simulink model "Modell_Diagnose"  (R2022a)
settings: Solver=FixedStepAuto  StartTime=0.0  StopTime=20.05  FixedStep=0.01  RelTol=1e-3
model workspace (MAT data in the model file):
  t_f = 7.2
libraries: simulink x3, fuzblock x1
settings Model: ParameterArgumentNames=t_f  Creator=Xueyong Lu  LastModifiedBy=Xueyong Lu

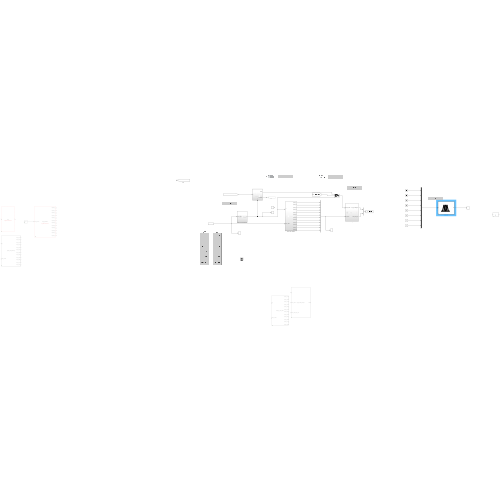
[thumbnail: Simulink's stored preview of the top-level diagram]
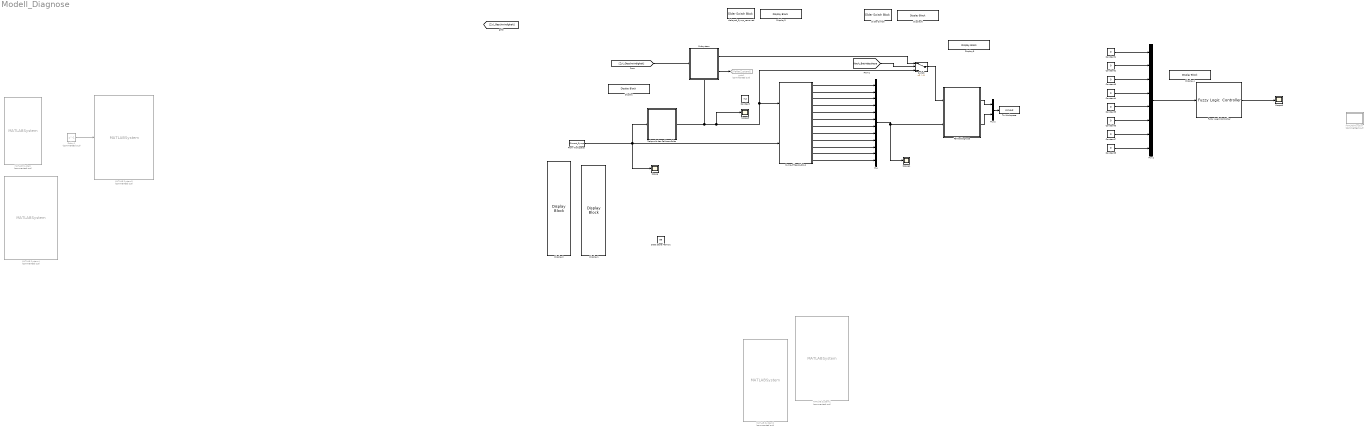
== system Modell_Diagnose ==
  Constant : Constant  Value=7.2  SampleTime=-1
  Constant{1..8} (8 alike) : Constant  Value=0
  Data Store Memory : DataStoreMemory  DataStoreName=aa  WriteAfterWriteMsg=warning  ShowAdditionalParam=off
  Delay1 : Delay  Commented=on  DelayLength=1
  Display{,3..6} (5 alike) : DisplayBlock  LabelPosition=Hide  Transparency=1
  Display1 : DisplayBlock  Transparency=1
  Display2 : DisplayBlock  Transparency=1  Layout=Fill available space
  Fehlerdiagnose : Subsystem
  From Workspace : FromWorkspace  VariableName=Simout_Symp  OutDataTypeStr=double  SampleTime=-1  OutputAfterFinalValue=Holding final value
  Fuzzy Logic Controller : fuzblock/Fuzzy Logic  Controller  FIS='Diagnose_fis_Still_Seite_A.fis'  OutputSampleNumber=101  DataType=double  FuzzifiedInputs=off  RuleFiringStrengths=off  RuleOutputs=off  AggregatedOutputs=off  SimulateUsing=Interpreted execution  OutOfRangeInputValueMessage=warning  NoRuleFiredMessage=warning  EmptyOutputFuzzySetMessage=warning
  MATLAB Function : MATLAB Function  Commented=on  TreatAsAtomicUnit=on
  MATLAB System : MATLABSystem  Commented=on  System=test  SimulateUsing=Code generation
      mask Type: test
      mask Display:
      | disp('test');
      | port_label('input',1,'u');
      | port_label('output',1,'y');
  MATLAB System1 : MATLABSystem  Commented=on  System=Symp_Filter_SubSys  SimulateUsing=Code generation
      mask Type: Symp_Filter_SubSys
      mask Display:
      | disp('Symp_Filter_SubSys');
      | port_label('input',1,'t_f');
      | port_label('input',2,'Time_series');
      | port_label('input',3,'Time_series_dis_der');
      | port_label('output',1,'Out');
  MATLAB System2 : MATLABSystem  Commented=on  System=output_in_eval_time  SimulateUsing=Code generation
      mask Type: output_in_eval_time
      mask Display:
      | disp('output_in_eval_time');
      | port_label('input',1,'t_f');
      | port_label('input',2,'Time_series');
      | port_label('output',1,'Symp_A1');
      | port_label('output',2,'Symp_A2');
      | port_label('output',3,'Symp_A3');
      | port_label('output',4,'Symp_A4');
      | port_label('output',5,'Symp_A5');
      | port_label('output',6,'Symp_B1');
      | port_label('output',7,'Symp_B2');
      | port_label('output',8,'Symp_B3');
      | port_label('output',9,'Symp_B4');
      | port_label('output',10,'Symp_B5');
      | port_label('output',11,'Symp_S1');
      | port_label('output',12,'Symp_S2');
  MATLAB System3 : MATLABSystem  Commented=on  System=Signal_Demux  SimulateUsing=Code generation
      mask Type: Signal_Demux
      mask Display:
      | disp('Signal_Demux');
      | port_label('input',1,'Time_series');
      | port_label('output',1,'Symp_A1');
      | port_label('output',2,'Symp_A2');
      | port_label('output',3,'Symp_A3');
      | port_label('output',4,'Symp_A4');
      | port_label('output',5,'Symp_A5');
      | port_label('output',6,'Symp_B1');
      | port_label('output',7,'Symp_B2');
      | port_label('output',8,'Symp_B3');
      | port_label('output',9,'Symp_B4');
      | port_label('output',10,'Symp_B5');
      | port_label('output',11,'Symp_S1');
      | port_label('output',12,'Symp_S2');
  MATLAB System4 : MATLABSystem  Commented=on  System=Symp_Filter_SubSys  SimulateUsing=Code generation
      mask Type: Symp_Filter_SubSys
      mask Display:
      | disp('Symp_Filter_SubSys');
      | port_label('input',1,'t_f');
      | port_label('input',2,'Time_series');
      | port_label('output',1,'Symp_A1');
      | port_label('output',2,'Symp_A2');
      | port_label('output',3,'Symp_A3');
      | port_label('output',4,'Symp_A4');
      | port_label('output',5,'Symp_A5');
      | port_label('output',6,'Symp_B1');
      | port_label('output',7,'Symp_B2');
      | port_label('output',8,'Symp_B3');
      | port_label('output',9,'Symp_B4');
      | port_label('output',10,'Symp_B5');
      | port_label('output',11,'Symp_S1');
      | port_label('output',12,'Symp_S2');
  Mux : Mux  Inputs=12
  Mux1 : Mux  Inputs=8
  Mux2 : Mux  Inputs=2
  Scope{,1,3,5} (4 alike) : Scope
  Slider Switch : SliderSwitchBlock
      settings: Values={{'Nach_t_f', 'Nach_vZyl'}, [0 1]}
  Subsystem : Subsystem
      settings: PortSchema="{\"entries\":[{\"content\":{\"sides\":[{\"content\":{\"connectorIds\":[\"In1\"]},\"type\":\"ConnectorPlacement.EquallySpacedRectSide\",\"uuid\":\"f9972d87-f39c-4f1f-a94a-1eb1a94210bf\"},{\"content\":{\"connectorIds\":[\"Out1\",\"Out2\"],\"side\":\"RIGHT\"},\"type\":\"ConnectorPlacement.EquallySpacedRectSide\",\"uuid\":\"518922ff-8880-4fb1-9f47-52b625cdf1df\"},{\"content\":{\"connectorIds\":[],\"side\":\"TOP\"},\"type\":\"ConnectorPlacement.EquallySpacedRectSide\",\"uuid\":\"62199aae-54b7-4722-ae08-096fbd9bf566\"},{\"content\":{\"connectorIds\":[\"In2\"],\"side\":\"BOTTOM\"},\"type\":\"ConnectorPlacement.EquallySpacedRectSide\",\"uuid\":\"39e1fdf6-478a-4c85-b443-9280ada7e399\"}]},\"type\":\"ConnectorPlacement.EquallySpacedConnector\",\"uuid\":\"c265ec14-a46e-406d-bb29-39e6e28d34ef\"}],\"packageUris\":[\"http://schema.mathworks.com/mf0/Connector/R2020b\"],\"version\":\"1.0\"}"
  Switch : Switch  Criteria=u2 > Threshold  SaturateOnIntegerOverflow=off  InputSameDT=off
  Symp_Filter_SubSys : Subsystem
  To Workspace : ToWorkspace  VariableName=simout  SaveFormat=Timeseries  SampleTime=-1
  Zeitpunkt des Fehlerauftritts : Subsystem
  delayed_Symp_removed : SliderSwitchBlock
      settings: Values={{'Off', 'On'}, [0 1]}
  goto1 : Goto  Commented=on  GotoTag=FehlerZustand
  wires:
  Symp_Filter_SubSys/1(Symp_A1) -> Mux/1
  Symp_Filter_SubSys/2(Symp_A2) -> Mux/2
  Symp_Filter_SubSys/3(Symp_A3) -> Mux/3
  Symp_Filter_SubSys/4(Symp_A4) -> Mux/4
  Symp_Filter_SubSys/5(Symp_A5) -> Mux/5
  Symp_Filter_SubSys/6(Symp_B1) -> Mux/6
  Symp_Filter_SubSys/7(Symp_B2) -> Mux/7
  Symp_Filter_SubSys/8(Symp_B3) -> Mux/8
  Symp_Filter_SubSys/9(Symp_B4) -> Mux/9
  Symp_Filter_SubSys/10(Symp_B5) -> Mux/10
  Symp_Filter_SubSys/11(Symp_S1) -> Mux/11
  Symp_Filter_SubSys/12(Symp_S2) -> Mux/12
  Delay1/1 -> MATLAB System3/1
  From Workspace/1 -> Zeitpunkt des Fehlerauftritts/1(Symp_matrix), Symp_Filter_SubSys/2(Symp_series), Scope/1
  Zeitpunkt des Fehlerauftritts/1(t_f) -> Subsystem/2(t_f), Scope3/1, Symp_Filter_SubSys/1(t_f), Switch/3
  Mux/1 -> Scope1/1, Fehlerdiagnose/2(Symptome)
  Constant8/1 -> Mux1/8
  Constant7/1 -> Mux1/7
  Constant6/1 -> Mux1/6
  Constant5/1 -> Mux1/5
  Constant4/1 -> Mux1/4
  Constant3/1 -> Mux1/3
  Constant2/1 -> Mux1/2
  Constant1/1 -> Mux1/1
  Mux1/1 -> Fuzzy Logic Controller/1
  Fuzzy Logic Controller/1 -> Scope5/1
  [Zyl_Geschwindigkeit] -> Subsystem/1(In1)
  Subsystem/2(FaultState) -> goto1/1
  Switch/1 -> Fehlerdiagnose/1(Fehler_Phase)
  [Nach_Betriebsphase] -> Switch/2
  Subsystem/1(Phase) -> Switch/1
  Fehlerdiagnose/1(Symp_zurDiagnose) -> Mux2/1
  Fehlerdiagnose/2(Fehler_komp_Nr) -> Mux2/2
  Mux2/1 -> To Workspace/1

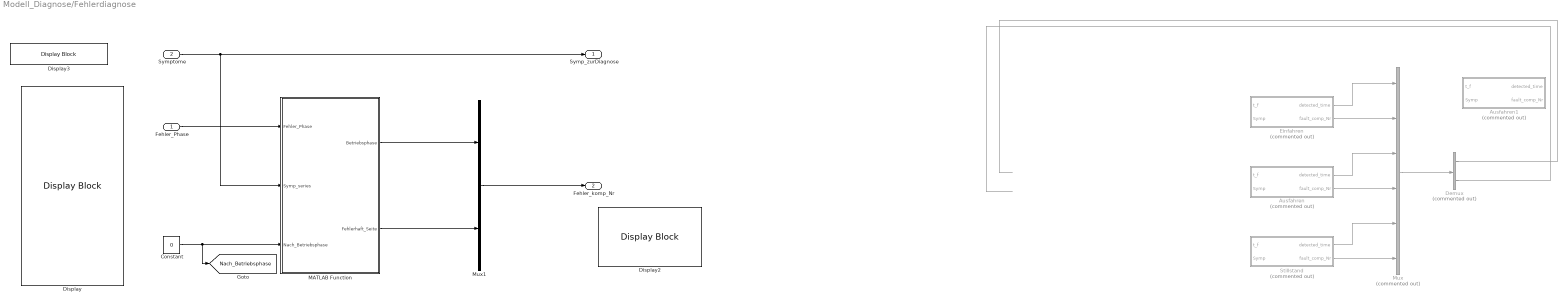
== system Modell_Diagnose/Fehlerdiagnose ==
  Fehler_Phase : Inport
  Symptome : Inport  Port=2
  Ausfahren : Subsystem  Commented=on
  Ausfahren1 : Subsystem  Commented=on
  Constant : Constant  Value=0
  Demux : Demux  Commented=on  Outputs=2
  Display : DisplayBlock  LabelPosition=Hide  Format=long  Transparency=1  Layout=Fill available space
  Display2 : DisplayBlock  LabelPosition=Hide  Transparency=1
  Display3 : DisplayBlock  LabelPosition=Hide  Transparency=1
  Einfahren : Subsystem  Commented=on
  MATLAB Function : MATLAB Function  TreatAsAtomicUnit=on
  Mux : Mux  Commented=on  Inputs=6
  Mux1 : Mux  Inputs=2
  Stillstand : Subsystem  Commented=on
  Symp_zurDiagnose : Outport
  Fehler_komp_Nr : Outport  Port=2
  tag scope: Nach_Betriebsphase=global
  wires:
  ? -> Einfahren/1(t_f)
  ? -> Ausfahren/1(t_f)
  ? -> Stillstand/1(t_f)
  Einfahren/1(detected_time) -> Mux/1
  Mux/1 -> Demux/1
  Einfahren/2(fault_comp_Nr) -> Mux/2
  Ausfahren/1(detected_time) -> Mux/3
  Ausfahren/2(fault_comp_Nr) -> Mux/4
  Stillstand/1(detected_time) -> Mux/5
  Stillstand/2(fault_comp_Nr) -> Mux/6
  Demux/1 -> ?
  Demux/2 -> ?
  Constant/1 -> MATLAB Function/3(Nach_Betriebsphase), [Nach_Betriebsphase]
  Fehler_Phase/1 -> MATLAB Function/1(Fehler_Phase)
  Mux1/1 -> Fehler_komp_Nr/1
  Symptome/1 -> MATLAB Function/2(Symp_series), Symp_zurDiagnose/1
  MATLAB Function/1(Betriebsphase) -> Mux1/1
  MATLAB Function/2(Fehlerhaft_Seite) -> Mux1/2

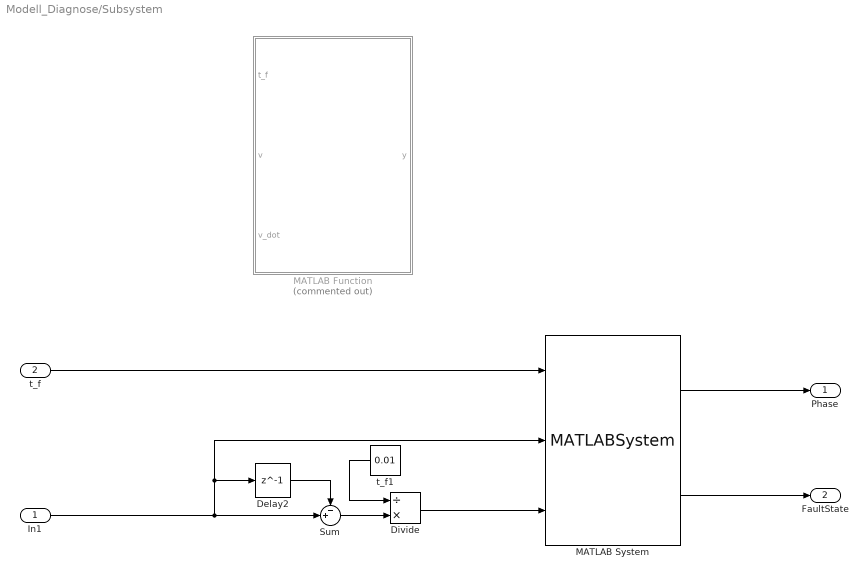
== system Modell_Diagnose/Subsystem ==
  In1 : Inport
  t_f : Inport  Port=2
  Delay2 : Delay  DelayLength=1
  Divide : Product  Inputs=/*
  MATLAB Function : MATLAB Function  Commented=on  TreatAsAtomicUnit=on
  MATLAB System : MATLABSystem  System=Betriebs_Phase  SimulateUsing=Code generation
      mask Type: Betriebs_Phase
      mask Display:
      | disp('Betriebs_Phase');
      | port_label('input',1,'t_f');
      | port_label('input',2,'v');
      | port_label('input',3,'v_dot');
      | port_label('output',1,'Phase');
      | port_label('output',2,'Fault_State');
  Sum : Sum  Inputs=-+|
  t_f1 : Constant  Value=0.01  VectorParams1D=off
  Phase : Outport
  FaultState : Outport  Port=2
  wires:
  In1/1 -> MATLAB System/2, Delay2/1, Sum/2
  t_f1/1 -> Divide/1
  Sum/1 -> Divide/2
  Delay2/1 -> Sum/1
  Divide/1 -> MATLAB System/3
  t_f/1 -> MATLAB System/1
  MATLAB System/1 -> Phase/1
  MATLAB System/2 -> FaultState/1

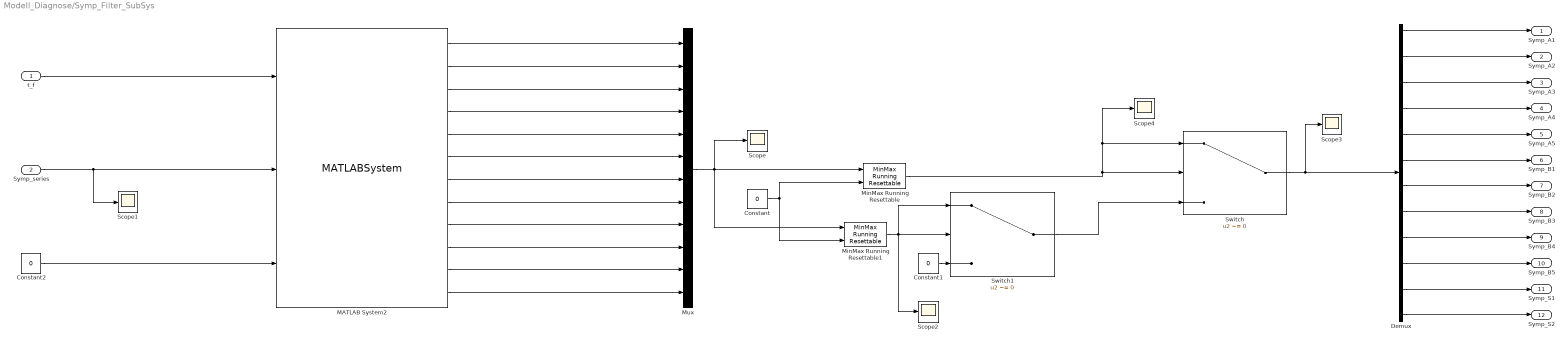
== system Modell_Diagnose/Symp_Filter_SubSys ==
  t_f : Inport
  Symp_series : Inport  Port=2
  Constant : Constant  Value=0  OutDataTypeStr=boolean
  Constant1 : Constant  Value=0  OutDataTypeStr=boolean
  Constant2 : Constant  Value=0
  Demux : Demux  Outputs=12
  MATLAB System2 : MATLABSystem  System=output_in_eval_time  SimulateUsing=Code generation
      mask Type: output_in_eval_time
      mask Display:
      | disp('output_in_eval_time');
      | port_label('input',1,'t_f');
      | port_label('input',2,'Symp_series');
      | port_label('input',3,'delayed_Symp_removed');
      | port_label('output',1,'Symp_A1');
      | port_label('output',2,'Symp_A2');
      | port_label('output',3,'Symp_A3');
      | port_label('output',4,'Symp_A4');
      | port_label('output',5,'Symp_A5');
      | port_label('output',6,'Symp_B1');
      | port_label('output',7,'Symp_B2');
      | port_label('output',8,'Symp_B3');
      | port_label('output',9,'Symp_B4');
      | port_label('output',10,'Symp_B5');
      | port_label('output',11,'Symp_S1');
      | port_label('output',12,'Symp_S2');
  MinMax Running Resettable : simulink/Math Operations/MinMax Running Resettable  Function=max  vinit=0.0
  MinMax Running Resettable1 : simulink/Math Operations/MinMax Running Resettable  Function=min  vinit=0.0
  Mux : Mux  Inputs=12
  Scope{,1..4} (5 alike) : Scope
  Switch : Switch  Criteria=u2 ~= 0  SaturateOnIntegerOverflow=off  InputSameDT=off
  Switch1 : Switch  Criteria=u2 ~= 0  SaturateOnIntegerOverflow=off  InputSameDT=off
  Symp_A1 : Outport
  Symp_A2 : Outport  Port=2
  Symp_A3 : Outport  Port=3
  Symp_A4 : Outport  Port=4
  Symp_A5 : Outport  Port=5
  Symp_B1 : Outport  Port=6
  Symp_B2 : Outport  Port=7
  Symp_B3 : Outport  Port=8
  Symp_B4 : Outport  Port=9
  Symp_B5 : Outport  Port=10
  Symp_S1 : Outport  Port=11
  Symp_S2 : Outport  Port=12
  wires:
  Symp_series/1 -> Scope1/1, MATLAB System2/2
  MATLAB System2/1 -> Mux/1
  MATLAB System2/2 -> Mux/2
  MATLAB System2/3 -> Mux/3
  MATLAB System2/4 -> Mux/4
  MATLAB System2/5 -> Mux/5
  MATLAB System2/6 -> Mux/6
  MATLAB System2/7 -> Mux/7
  MATLAB System2/8 -> Mux/8
  MATLAB System2/9 -> Mux/9
  MATLAB System2/10 -> Mux/10
  MATLAB System2/11 -> Mux/11
  MATLAB System2/12 -> Mux/12
  MinMax Running Resettable1/1 -> Scope2/1, Switch1/1, Switch1/2
  Switch/1 -> Scope3/1, Demux/1
  Mux/1 -> Scope/1, MinMax Running Resettable/1, MinMax Running Resettable1/1
  MinMax Running Resettable/1 -> Switch/1, Scope4/1, Switch/2
  Constant/1 -> MinMax Running Resettable1/2, MinMax Running Resettable/2
  Switch1/1 -> Switch/3
  Constant1/1 -> Switch1/3
  Demux/1 -> Symp_A1/1
  Demux/2 -> Symp_A2/1
  Demux/3 -> Symp_A3/1
  Demux/4 -> Symp_A4/1
  Demux/5 -> Symp_A5/1
  Demux/6 -> Symp_B1/1
  Demux/7 -> Symp_B2/1
  Demux/8 -> Symp_B3/1
  Demux/9 -> Symp_B4/1
  Demux/10 -> Symp_B5/1
  Demux/11 -> Symp_S1/1
  Demux/12 -> Symp_S2/1
  t_f/1 -> MATLAB System2/1
  Constant2/1 -> MATLAB System2/3

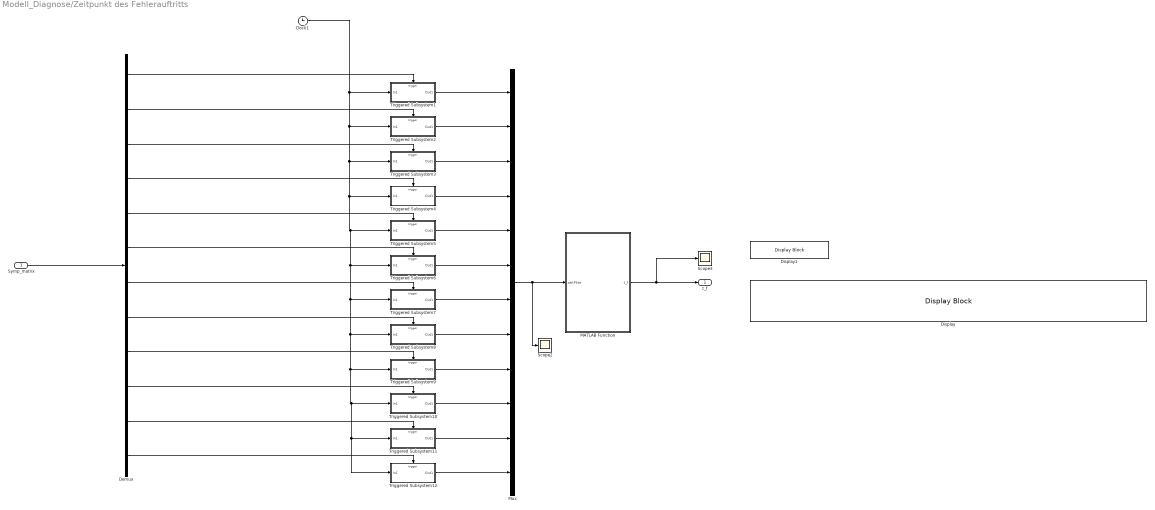
== system Modell_Diagnose/Zeitpunkt des Fehlerauftritts ==
  Symp_matrix : Inport
  Clock1 : Clock
  Demux : Demux  Outputs=12
  Display : DisplayBlock  LabelPosition=Hide  Transparency=1
  Display1 : DisplayBlock  LabelPosition=Hide  Transparency=1
  MATLAB Function : MATLAB Function  TreatAsAtomicUnit=on
  Mux : Mux  Inputs=12
  Scope2 : Scope
  Scope3 : Scope
  Triggered Subsystem1 : Subsystem  TreatAsAtomicUnit=on
  Triggered Subsystem10 : Subsystem  TreatAsAtomicUnit=on
  Triggered Subsystem11 : Subsystem  TreatAsAtomicUnit=on
  Triggered Subsystem12 : Subsystem  TreatAsAtomicUnit=on
  Triggered Subsystem2 : Subsystem  TreatAsAtomicUnit=on
  Triggered Subsystem3 : Subsystem  TreatAsAtomicUnit=on
  Triggered Subsystem4 : Subsystem  TreatAsAtomicUnit=on
  Triggered Subsystem5 : Subsystem  TreatAsAtomicUnit=on
  Triggered Subsystem6 : Subsystem  TreatAsAtomicUnit=on
  Triggered Subsystem7 : Subsystem  TreatAsAtomicUnit=on
  Triggered Subsystem8 : Subsystem  TreatAsAtomicUnit=on
  Triggered Subsystem9 : Subsystem  TreatAsAtomicUnit=on
  t_f : Outport
  wires:
  Demux/2 -> Triggered Subsystem2/Trigger
  Demux/1 -> Triggered Subsystem1/Trigger
  Demux/3 -> Triggered Subsystem3/Trigger
  Demux/4 -> Triggered Subsystem4/Trigger
  Demux/6 -> Triggered Subsystem6/Trigger
  Demux/5 -> Triggered Subsystem5/Trigger
  Demux/7 -> Triggered Subsystem7/Trigger
  Clock1/1 -> Triggered Subsystem4/1(In1), Triggered Subsystem12/1(In1), Triggered Subsystem11/1(In1), Triggered Subsystem10/1(In1), Triggered Subsystem9/1(In1), Triggered Subsystem8/1(In1), Triggered Subsystem7/1(In1), Triggered Subsystem6/1(In1), Triggered Subsystem5/1(In1), Triggered Subsystem3/1(In1), Triggered Subsystem2/1(In1), Triggered Subsystem1/1(In1)
  Triggered Subsystem1/1(Out1) -> Mux/1
  Symp_matrix/1 -> Demux/1
  Mux/1 -> Scope2/1, MATLAB Function/1(zeitPkte)
  MATLAB Function/1(t_f) -> Scope3/1, t_f/1
  Demux/8 -> Triggered Subsystem8/Trigger
  Demux/9 -> Triggered Subsystem9/Trigger
  Demux/10 -> Triggered Subsystem10/Trigger
  Demux/11 -> Triggered Subsystem11/Trigger
  Demux/12 -> Triggered Subsystem12/Trigger
  Triggered Subsystem12/1(Out1) -> Mux/12
  Triggered Subsystem2/1(Out1) -> Mux/2
  Triggered Subsystem3/1(Out1) -> Mux/3
  Triggered Subsystem4/1(Out1) -> Mux/4
  Triggered Subsystem5/1(Out1) -> Mux/5
  Triggered Subsystem6/1(Out1) -> Mux/6
  Triggered Subsystem7/1(Out1) -> Mux/7
  Triggered Subsystem8/1(Out1) -> Mux/8
  Triggered Subsystem9/1(Out1) -> Mux/9
  Triggered Subsystem10/1(Out1) -> Mux/10
  Triggered Subsystem11/1(Out1) -> Mux/11

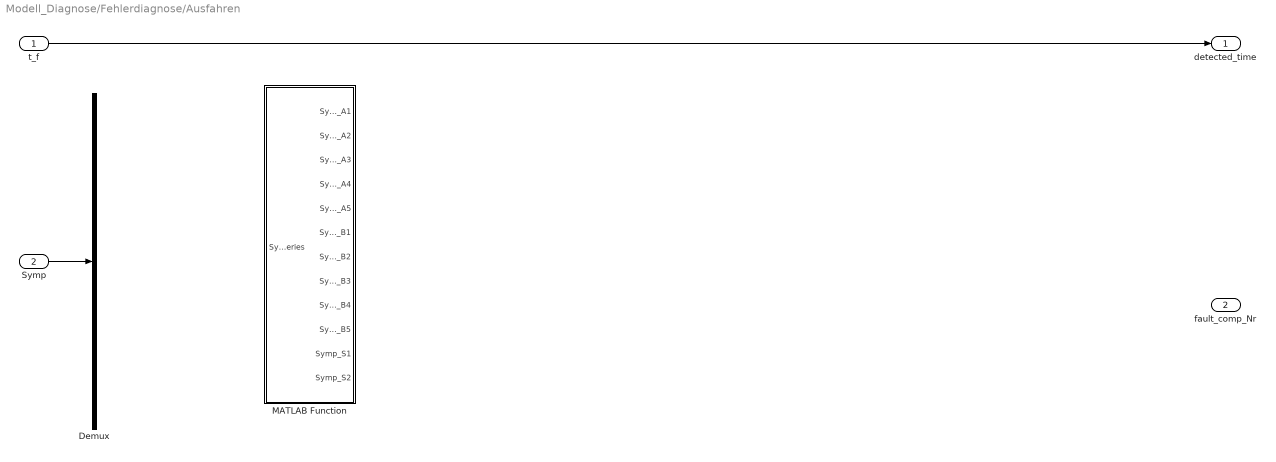
== system Modell_Diagnose/Fehlerdiagnose/Ausfahren ==
  t_f : Inport
  Symp : Inport  Port=2
  Demux : Demux  Outputs=12
  MATLAB Function : MATLAB Function  TreatAsAtomicUnit=on
  detected_time : Outport
  fault_comp_Nr : Outport  Port=2
  wires:
  Symp/1 -> Demux/1
  t_f/1 -> detected_time/1

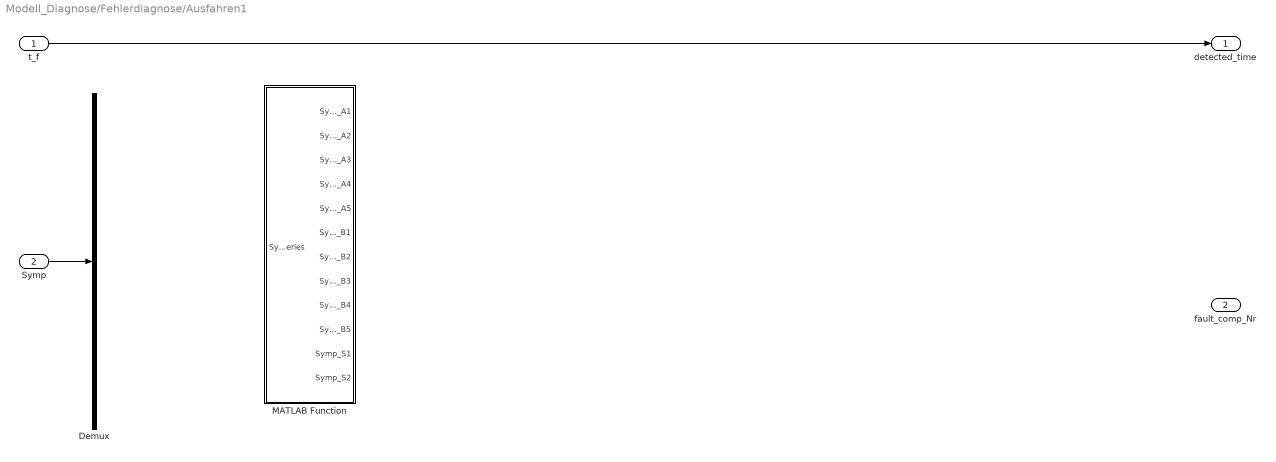
== system Modell_Diagnose/Fehlerdiagnose/Ausfahren1 ==
  t_f : Inport
  Symp : Inport  Port=2
  Demux : Demux  Outputs=12
  MATLAB Function : MATLAB Function  TreatAsAtomicUnit=on
  detected_time : Outport
  fault_comp_Nr : Outport  Port=2
  wires:
  Symp/1 -> Demux/1
  t_f/1 -> detected_time/1

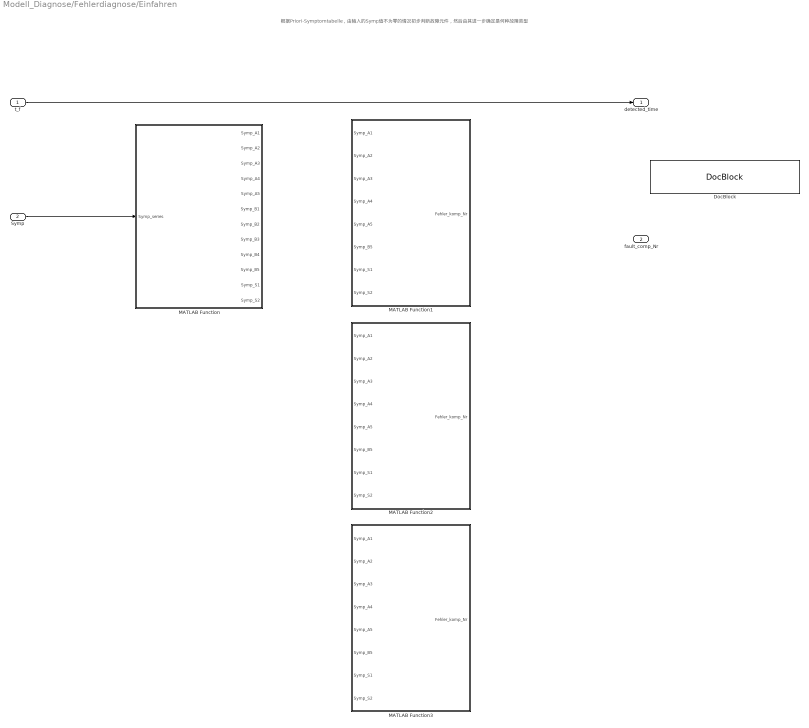
== system Modell_Diagnose/Fehlerdiagnose/Einfahren ==
  note: 根据Priori-Symptomtabelle，由输入的Symp值不为零的情况初步判断故障元件，然后由其进一步确定是何种故障类型
  t_f : Inport
  Symp : Inport  Port=2
  DocBlock : simulink/Model-Wide Utilities/DocBlock  DocumentType=Text
      content=|
      | 根据Priori-Symptomtabelle，由输入的Symp值不为零的情况初步判断故障元件，然后由其进一步确定是何种故障类型
  MATLAB Function : MATLAB Function  TreatAsAtomicUnit=on
  MATLAB Function1 : MATLAB Function  TreatAsAtomicUnit=on
  MATLAB Function2 : MATLAB Function  TreatAsAtomicUnit=on
  MATLAB Function3 : MATLAB Function  TreatAsAtomicUnit=on
  detected_time : Outport
  fault_comp_Nr : Outport  Port=2
  wires:
  Symp/1 -> MATLAB Function/1(Symp_series)
  t_f/1 -> detected_time/1

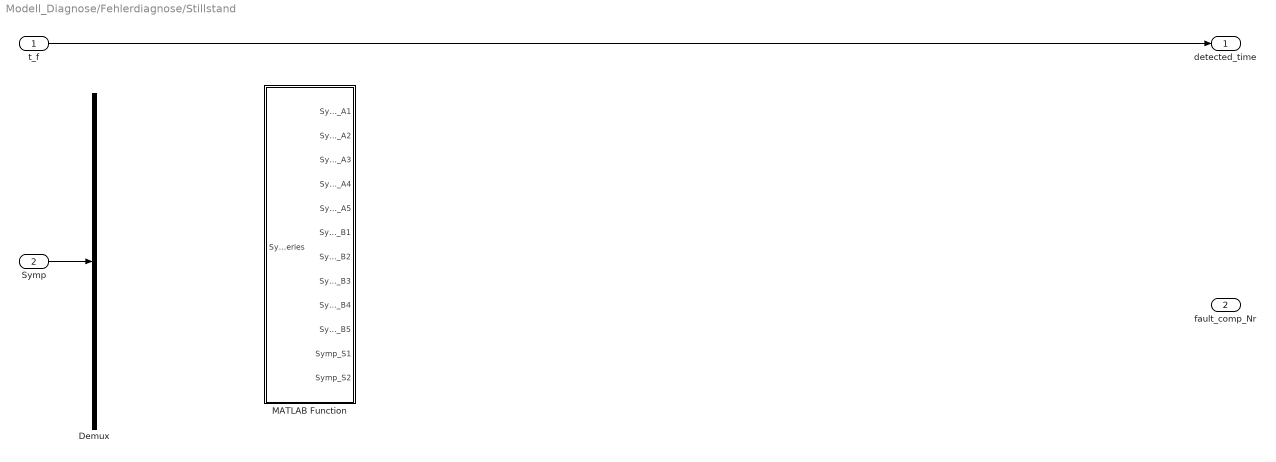
== system Modell_Diagnose/Fehlerdiagnose/Stillstand ==
  t_f : Inport
  Symp : Inport  Port=2
  Demux : Demux  Outputs=12
  MATLAB Function : MATLAB Function  TreatAsAtomicUnit=on
  detected_time : Outport
  fault_comp_Nr : Outport  Port=2
  wires:
  Symp/1 -> Demux/1
  t_f/1 -> detected_time/1

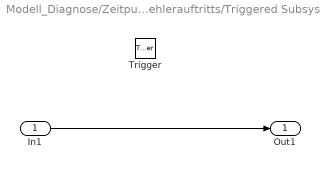
== system Modell_Diagnose/Zeitpunkt des Fehlerauftritts/Triggered Subsystem1 ==
  In1 : Inport
  Trigger : TriggerPort  TriggerType=either  VariantControl=(inherit)
  Out1 : Outport
  wires:
  In1/1 -> Out1/1

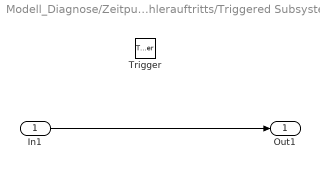
== system Modell_Diagnose/Zeitpunkt des Fehlerauftritts/Triggered Subsystem10 ==
  In1 : Inport
  Trigger : TriggerPort  TriggerType=either  VariantControl=(inherit)
  Out1 : Outport
  wires:
  In1/1 -> Out1/1

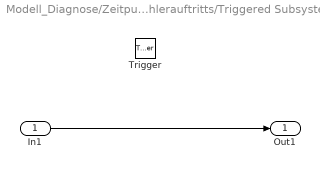
== system Modell_Diagnose/Zeitpunkt des Fehlerauftritts/Triggered Subsystem11 ==
  In1 : Inport
  Trigger : TriggerPort  TriggerType=either  VariantControl=(inherit)
  Out1 : Outport
  wires:
  In1/1 -> Out1/1

== system Modell_Diagnose/Zeitpunkt des Fehlerauftritts/Triggered Subsystem12 ==
  In1 : Inport
  Trigger : TriggerPort  TriggerType=either  VariantControl=(inherit)
  Out1 : Outport
  wires:
  In1/1 -> Out1/1

== system Modell_Diagnose/Zeitpunkt des Fehlerauftritts/Triggered Subsystem2 ==
  In1 : Inport
  Trigger : TriggerPort  TriggerType=either  VariantControl=(inherit)
  Out1 : Outport
  wires:
  In1/1 -> Out1/1

== system Modell_Diagnose/Zeitpunkt des Fehlerauftritts/Triggered Subsystem3 ==
  In1 : Inport
  Trigger : TriggerPort  TriggerType=either  VariantControl=(inherit)
  Out1 : Outport
  wires:
  In1/1 -> Out1/1

== system Modell_Diagnose/Zeitpunkt des Fehlerauftritts/Triggered Subsystem4 ==
  In1 : Inport
  Trigger : TriggerPort  TriggerType=either  VariantControl=(inherit)
  Out1 : Outport
  wires:
  In1/1 -> Out1/1

== system Modell_Diagnose/Zeitpunkt des Fehlerauftritts/Triggered Subsystem5 ==
  In1 : Inport
  Trigger : TriggerPort  TriggerType=either  VariantControl=(inherit)
  Out1 : Outport
  wires:
  In1/1 -> Out1/1

== system Modell_Diagnose/Zeitpunkt des Fehlerauftritts/Triggered Subsystem6 ==
  In1 : Inport
  Trigger : TriggerPort  TriggerType=either  VariantControl=(inherit)
  Out1 : Outport
  wires:
  In1/1 -> Out1/1

== system Modell_Diagnose/Zeitpunkt des Fehlerauftritts/Triggered Subsystem7 ==
  In1 : Inport
  Trigger : TriggerPort  TriggerType=either  VariantControl=(inherit)
  Out1 : Outport
  wires:
  In1/1 -> Out1/1

== system Modell_Diagnose/Zeitpunkt des Fehlerauftritts/Triggered Subsystem8 ==
  In1 : Inport
  Trigger : TriggerPort  TriggerType=either  VariantControl=(inherit)
  Out1 : Outport
  wires:
  In1/1 -> Out1/1

== system Modell_Diagnose/Zeitpunkt des Fehlerauftritts/Triggered Subsystem9 ==
  In1 : Inport
  Trigger : TriggerPort  TriggerType=either  VariantControl=(inherit)
  Out1 : Outport
  wires:
  In1/1 -> Out1/1

== matlab function Modell_Diagnose/Fehlerdiagnose/Einfahren/MATLAB Function1 ==
  data: Fehler_komp_Nr output; Symp_A1 input; Symp_A2 input; Symp_A3 input; Symp_A4 input; Symp_A5 input; Symp_B5 input; Symp_S1 input; Symp_S2 input
function Fehler_komp_Nr = Einfahren_Seite_A(Symp_A1,Symp_A2,Symp_A3,Symp_A4,Symp_A5,Symp_B5,Symp_S1,Symp_S2)

== matlab function Modell_Diagnose/Fehlerdiagnose/Einfahren/MATLAB Function2 ==
  data: Fehler_komp_Nr output; Symp_A1 input; Symp_A2 input; Symp_A3 input; Symp_A4 input; Symp_A5 input; Symp_B5 input; Symp_S1 input; Symp_S2 input
function Fehler_komp_Nr = Einfahren_Seite_B(Symp_A1,Symp_A2,Symp_A3,Symp_A4,Symp_A5,Symp_B5,Symp_S1,Symp_S2)

== matlab function Modell_Diagnose/Fehlerdiagnose/Einfahren/MATLAB Function3 ==
  data: Fehler_komp_Nr output; Symp_A1 input; Symp_A2 input; Symp_A3 input; Symp_A4 input; Symp_A5 input; Symp_B5 input; Symp_S1 input; Symp_S2 input
function Fehler_komp_Nr = Einfahren_Seite_S(Symp_A1,Symp_A2,Symp_A3,Symp_A4,Symp_A5,Symp_B5,Symp_S1,Symp_S2)

== matlab function Modell_Diagnose/Fehlerdiagnose/Ausfahren1/MATLAB Function ==
  data: Symp_A1 output; Symp_series input; Symp_A2 output; Symp_A3 output; Symp_A4 output; Symp_A5 output; Symp_B1 output; Symp_B2 output; Symp_B3 output; Symp_B4 output; Symp_B5 output; Symp_S1 output; Symp_S2 output
function [Symp_A1,Symp_A2,Symp_A3,Symp_A4,Symp_A5,Symp_B1,Symp_B2,Symp_B3,Symp_B4,Symp_B5,Symp_S1,Symp_S2] = fcn(Symp_series)
    
y = u;

== matlab function Modell_Diagnose/Subsystem/MATLAB Function ==
  data: t_f input; v input; y output; v_dot input
function y = Betriebs_Phase1(t_f,v,v_dot)
    if v < 0
        if v_dot < 0
            y = 1;
        elseif v_dot == 0
            y = 2;
        else 
            y = 3;
        end
    elseif v > 0
        if v_dot > 0
            y = 5;
        elseif v_dot == 0
            y = 6;
        else
            y=7;
        end
    else
        if v_dot == 0
            y = 4;
        end
    end

== matlab function Modell_Diagnose/Fehlerdiagnose/MATLAB Function ==
  settings: updateMethod=DISCRETE
  data: Betriebsphase output; Fehlerhaft_Seite output; Fehler_Phase input; Symp_series input; Nach_Betriebsphase input
function [Betriebsphase,Fehlerhaft_Seite] = fcn(Fehler_Phase,Symp_series,Nach_Betriebsphase)
%% Ermittlung der Betriebsphase des Fehlerauftritts
Betriebsphase = nan;  % Initialisierung der Ausgangsgrößen
Fehlerhaft_Seite = nan;

if logical(Nach_Betriebsphase)
%     case 1
        if Fehler_Phase == 1 || Fehler_Phase == 2 || Fehler_Phase == 3
            Betriebsphase = 1; % Einfahren
        elseif Fehler_Phase == 5 || Fehler_Phase == 6 || Fehler_Phase == 7
            Betriebsphase = 2; % Ausfahren
        elseif Fehler_Phase == 4
            Betriebsphase = 3; % Stillstand
        end
%     case 0
else
        if Fehler_Phase < 12
            Betriebsphase = 1; % Einfahren
        elseif Fehler_Phase > 14 && Fehler_Phase < 20
            Betriebsphase = 2; % Ausfahren
        elseif Fehler_Phase == 20
            Betriebsphase = 0;
        else
            Betriebsphase = 3; % Stillstand
        end
end
%% Lokalisierung der fehlerhaften Seite
switch Betriebsphase
    %% Phase der Fehlererkennung: Einfahren
    % A:1, B:2, S:3, unerkennbar A-P,B-T: 4, unerkennbar A-T, B-P: 5 
    case 1
    if all(Symp_series==0)
        Fehlerhaft_Seite = 0;

    elseif all(Symp_series(1:9)==0)   % A1-B4
        if Symp_series(10)==0         % B5 == 0
            if all(Symp_series(11:12) < 0)  % S1-S2
                Fehlerhaft_Seite = 1; % A-P_min
            elseif all(Symp_series(11:12) > 0)
                Fehlerhaft_Seite = 5; % A-T_max, B-P_max, p0_sens
            elseif Symp_series(11)<0 && Symp_series(12)==0
                Fehlerhaft_Seite = 1; % pA_sens
            elseif Symp_series(11) == 0 && Symp_series(12) > 0
                Fehlerhaft_Seite = 3; % p0_sens
            end
        elseif Symp_series(10) > 0    % B5 > 0
            if all(Symp_series(11:12) < 0)
                Fehlerhaft_Seite = 4; % A-P_max, B-T_max
            elseif all(Symp_series(11:12) == 0)
                Fehlerhaft_Seite = 2; % B-T_max
            end
        elseif Symp_series(10) < 0    % B5 < 0
            if all(Symp_series(11:12) > 0)
                Fehlerhaft_Seite = 3; % p0_sens
            end
        end

    elseif length(find(Symp_series(1:5)~=0)) > length(find(Symp_series(6:10)~=0))...
            && length(find(Symp_series(6:10)~=0))<=1                       % Symptome auf der Seite_A > die auf der Seite_B
        [A_NonNull_Nr,NonNull_ind] = find(Symp_series(1:5)~=0);
        switch length(A_NonNull_Nr)
            case 1
                if NonNull_ind(1) == 1
                    if all(Symp_series(2:12) == 0)
                        Fehlerhaft_Seite = 6; % --> swA-T, p0_sens, pT_sens; Eintragen in Seite S
                    else 
                        Fehlerhaft_Seite = 3;
                    end
                elseif NonNull_ind(1) == 4
                    if ~all(Symp_series(2:12) == 0)
                        Fehlerhaft_Seite = 3; % vZyl
                    else
                        Fehlerhaft_Seite = 1;
                    end
                else
                    Fehlerhaft_Seite = 1;
                end

            case 2 
                if all(NonNull_ind == [1 4])
                    Fehlerhaft_Seite = 3; % vZyl_sens
                elseif all(NonNull_ind == [3 4])
                    Fehlerhaft_Seite = 7; % vZyl_sens, pGSK_A, p_A_sens --> Eintragen in Seite A
                else
                    Fehlerhaft_Seite = 1;
%                     Symp_Vektor = Symp_series([1:5 10 11:12]);
                end

            case 3
                if all(NonNull_ind == [1 3 4])
                    Fehlerhaft_Seite = 8; % vZyl_sens, pA_sens --> Eintragen in Seite A (1)
                else
                    Fehlerhaft_Seite = 1;
                end

            case 4
                Fehlerhaft_Seite = 1;
        end

%         Symp_Vektor = Symp_series()
    
    elseif length(find(Symp_series(1:5)~=0)) <= length(find(Symp_series(6:10)~=0))...
            && length(find(Symp_series(1:5)~=0))<=1                       % Symptome auf der Seite_B >= die auf der Seite_A

        [A_NonNull_Nr,NonNull_ind] = find(Symp_series(6:10)~=0);
        switch length(A_NonNull_Nr)
            case 1
                if NonNull_ind(1) == 6
                    if all(Symp_series([1:5 11:12])==0)
                        Fehlerhaft_Seite = 8; % p0_sens, sw_B-P_min --> Eintragen in Seite B (2)
                    elseif Symp_series(1)~=0
                        Fehlerhaft_Seite = 1;
                    else
                        Fehlerhaft_Seite = 3;
                    end
                elseif NonNull_ind(1) == 10
                    if all(Symp_series(1:5)==0)
                        Fehlerhaft_Seite = 3;
                    else
                        Fehlerhaft_Seite = 2;
                    end
                end

            case 2
                if all(NonNull_ind==[6 10])
                    if all(Symp_series(11:12)~=0)
                        Fehlerhaft_Seite = 3;
                    else
                        Fehlerhaft_Seite = 2;
                    end
                else
                    Fehlerhaft_Seite = 2;
                end

%             case 3
%                 Fehlerhaft_Seite = 2; % nB=3, (nB>=nA && nA<=1) nicht erfuellt
% 
%             case 4
%                 Fehlerhaft_Seite = 2; % nB=4, (nB>=nA && nA<=1) nicht erfuellt
% 
%             case 5
%                 Fehlerhaft_Seite = 2; % aus globaler Betrachtung des Systems ist B2 bzw. A2 immer gleich null

            otherwise
                Fehlerhaft_Seite = 2;

        end
    else
        Fehlerhaft_Seite = 3;
        
    end


    %% Phase der Fehlererkennung: Ausfahren
    % A:1, B:2, S:3, 
    case 2
    if all(Symp_series==0)
        Fehlerhaft_Seite = 0;

    elseif all(Symp_series(1:10)==0)   % nur S1 und S2
        [A_NonNull_Nr,~] = find(Symp_series(11:12)~=0);
        switch length(A_NonNull_Nr)
            case 1
                Fehlerhaft_Seite = 3;
            case 2
                if all(Symp_series(11:12)>0)
                    Fehlerhaft_Seite = 4;
                else
                    Fehlerhaft_Seite = 1;
                end
        end
    elseif length(find(Symp_series(1:5)~=0)) > length(find(Symp_series(6:10)~=0))...
            && length(find(Symp_series(6:10)~=0))<=1                       % Symptome auf der Seite_A > die auf der Seite_B
        [A_NonNull_Nr,NonNull_ind] = find(Symp_series(1:5)~=0);
        switch length(A_NonNull_Nr)
            case 1
                if NonNull_ind(1) == 1
                    if all(Symp_series(11:12)==0)
                        if Symp_series(1) > 0
                            Fehlerhaft_Seite = 3; % p0_sens
                        else
                            Fehlerhaft_Seite = 9; % sw-A-P_min und p0_sens
                        end
                    elseif all(Symp_series(11:12)<0)
                        Fehlerhaft_Seite = 9; % sw-A-P_min und p0_sens_max
                    else
                        Fehlerhaft_Seite = 3;
                    end
                elseif NonNull_ind(1) == 4
                    if all(Symp_series(11:12)==0)
                        if Symp_series(4) > 0
                            Fehlerhaft_Seite = 3; % vZyl
                        else
                            Fehlerhaft_Seite = 7; % vZyl_sens, pGSK_A, p_A_sens
                        end
                    else
                        Fehlerhaft_Seite = 3; % vZyl
                    end
                else
                    Fehlerhaft_Seite = 1;
                end

            case 2
                if all(NonNull_ind == [1 4])
                    Fehlerhaft_Seite = 8; % pA_sens, vZyl_add
                elseif all(NonNull_ind == [3 4])
                    if all(Symp_series(6:12) == 0)
                        Fehlerhaft_Seite = 10; % pGSK_A, vZyl_prop
                    else
                        Fehlerhaft_Seite = 3; % vZyl_prop
                    end
                else
                    Fehlerhaft_Seite = 1; 
                end


            case 3
                if all(NonNull_ind == [1 3 4])
                    if ~all(Symp_series(6:12) == 0)
                        Fehlerhaft_Seite = 3; % vZyl_sens_add
                    else
                        Fehlerhaft_Seite = 1;
                    end
                else
                    Fehlerhaft_Seite = 1;
                end

            otherwise
                Fehlerhaft_Seite = 1;
  
        end
    elseif length(find(Symp_series(1:5)~=0)) <= length(find(Symp_series(6:10)~=0))...
            && length(find(Symp_series(1:5)~=0))<=1                       % Symptome auf der Seite_A <= die auf der Seite_B
        [A_NonNull_Nr,NonNull_ind] = find(Symp_series(6:10)~=0);
        switch length(A_NonNull_Nr)
            case 1
                if NonNull_ind(1) == 2
                    Fehlerhaft_Seite = 2;
                else
                    Fehlerhaft_Seite = 11; % pT_sens.max, sw-B-T_min
                end

            otherwise
                Fehlerhaft_Seite = 2;
        end

    else
        Fehlerhaft_Seite = 3;


    end



    %% Phase der Fehlererkennung: Stillstand
    % A:1, B:2, S:3, 
    case 3
        if all(Symp_series==0)
        Fehlerhaft_Seite = 0;

        elseif all(Symp_series(1:10)==0)   % nur S1 und S2
        [A_NonNull_Nr,~] = find(Symp_series(11:12)~=0);
        switch length(A_NonNull_Nr)
            case 1
                Fehlerhaft_Seite = 3;  % p0_sens.min/null
            case 2
                if all(Symp_series(11:12)>0)
                    Fehlerhaft_Seite = 12; % sw-A-T_max, sw-B-P_max
                else
                    Fehlerhaft_Seite = 13; % sw-A-P_min, pB_sens.min/null
                end
        end


        elseif length(find(Symp_series(1:5)~=0)) > length(find(Symp_series(6:10)~=0))...
            && length(find(Symp_series(6:10)~=0))<=1                       % Symptome auf der Seite_A > die auf der Seite_B
            [A_NonNull_Nr,NonNull_ind] = find(Symp_series(1:5)~=0);
            switch length(A_NonNull_Nr)
                case 1
                    if NonNull_ind(1) == 1
                        Fehlerhaft_Seite = 3;
                    elseif NonNull_ind(1) == 4
                        if all(Symp_series(6:12)==0)
                            Fehlerhaft_Seite = 1;
                        else
                            Fehlerhaft_Seite = 3;
                        end
                    else
                        Fehlerhaft_Seite = 1;
                    end

                case 2
                    if all(NonNull_ind == [1 4])
                        Fehlerhaft_Seite = 8; % vZyl_sens, pA_sens
                    elseif all(NonNull_ind == [3 4])
                        if all(Symp_series(11:12)==0)
                            Fehlerhaft_Seite = 1; % pGSK_A
                        else
                            Fehlerhaft_Seite = 3; % vZyl
                        end
                    else
                        Fehlerhaft_Seite = 1; % yV_sens
                    end

                otherwise
                    Fehlerhaft_Seite = 1;

            end


        elseif length(find(Symp_series(1:5)~=0)) <= length(find(Symp_series(6:10)~=0))...
            && length(find(Symp_series(1:5)~=0))<=1                       % Symptome auf der Seite_A <= die auf der Seite_B
            [A_NonNull_Nr,NonNull_ind] = find(Symp_series(6:10)~=0);
            switch length(A_NonNull_Nr)
                case 1
                    if NonNull_ind(1) == 2
                        Fehlerhaft_Seite = 1;
                    else
                        Fehlerhaft_Seite = 3; % pT_sens
                    end

                otherwise
                    Fehlerhaft_Seite = 1;
            end

        else
            Fehlerhaft_Seite = 3;

        end




end
% 
% switch Fehlerhaft_Seite
%         case 1
%             Symp_Vektor = Symp_series([1:5 10 11:12]); % A1-A5, B5, S1-S2
% 
%         case 2
%             Symp_Vektor = Symp_series([5 6:10 11:12]); % A5, B1-B5, S1-S2
% 
%         case 3
%             Symp_Vektor = Symp_series;
% %         otherwise
% %             Symp_Vektor = zeros(1,12);
% end

== matlab function Modell_Diagnose/Zeitpunkt des Fehlerauftritts/MATLAB Function ==
  data: zeitPkte input; t_f output
function t_f = fcn(zeitPkte)
t_f = 20;
for i = 1:12
    if zeitPkte(i)~=0 && zeitPkte(i)<t_f
        t_f = zeitPkte(i);
    end
end

end

== matlab function Modell_Diagnose/MATLAB Function ==
  data: u input; y output
function y = fcn(u)

y = u;

== matlab function Modell_Diagnose/Fehlerdiagnose/Einfahren/MATLAB Function ==
  data: Symp_A1 output; Symp_series input; Symp_A2 output; Symp_A3 output; Symp_A4 output; Symp_A5 output; Symp_B1 output; Symp_B2 output; Symp_B3 output; Symp_B4 output; Symp_B5 output; Symp_S1 output; Symp_S2 output
function [Symp_A1,Symp_A2,Symp_A3,Symp_A4,Symp_A5,Symp_B1,Symp_B2,Symp_B3,Symp_B4,Symp_B5,Symp_S1,Symp_S2] = fcn(Symp_series)
    
y = u;

== matlab function Modell_Diagnose/Fehlerdiagnose/Ausfahren/MATLAB Function ==
  data: Symp_A1 output; Symp_series input; Symp_A2 output; Symp_A3 output; Symp_A4 output; Symp_A5 output; Symp_B1 output; Symp_B2 output; Symp_B3 output; Symp_B4 output; Symp_B5 output; Symp_S1 output; Symp_S2 output
function [Symp_A1,Symp_A2,Symp_A3,Symp_A4,Symp_A5,Symp_B1,Symp_B2,Symp_B3,Symp_B4,Symp_B5,Symp_S1,Symp_S2] = fcn(Symp_series)
    
y = u;

== matlab function Modell_Diagnose/Fehlerdiagnose/Stillstand/MATLAB Function ==
  data: Symp_A1 output; Symp_series input; Symp_A2 output; Symp_A3 output; Symp_A4 output; Symp_A5 output; Symp_B1 output; Symp_B2 output; Symp_B3 output; Symp_B4 output; Symp_B5 output; Symp_S1 output; Symp_S2 output
function [Symp_A1,Symp_A2,Symp_A3,Symp_A4,Symp_A5,Symp_B1,Symp_B2,Symp_B3,Symp_B4,Symp_B5,Symp_S1,Symp_S2] = fcn(Symp_series)
    
y = u;
